simulink model "Wind_Turbine_Modelling"  (R2025a)
settings: Solver=ode23tb  StartTime=0.0  StopTime=1  MaxStep=1e-4  RelTol=1e-3
libraries: simulink x1
settings Model: Creator=Jawad  LastModifiedBy=Jawad

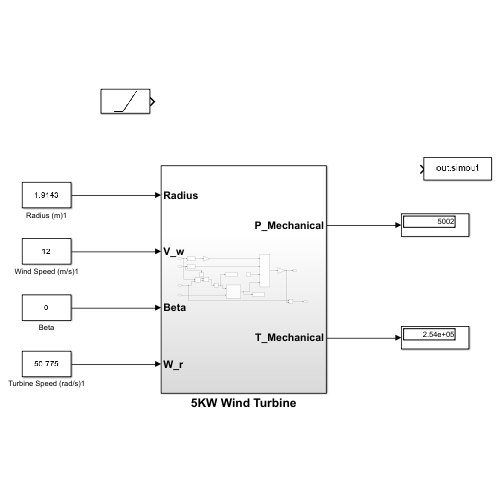
[thumbnail: Simulink's stored preview of the top-level diagram]
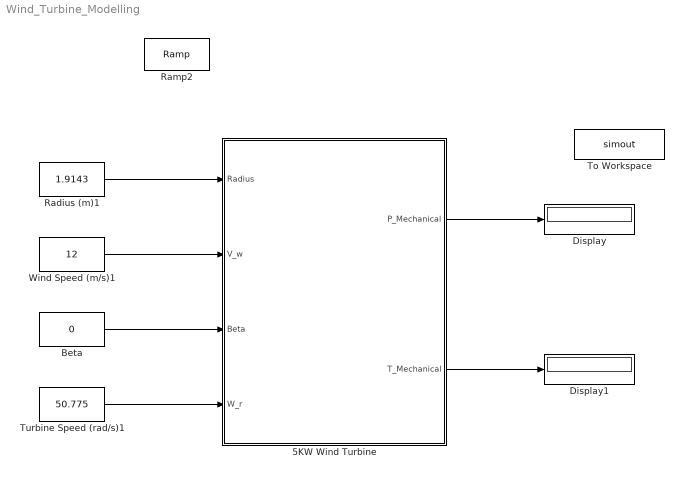
== system Wind_Turbine_Modelling ==
  5KW Wind Turbine : Subsystem
  Beta : Constant  Value=0
  Display : Display
  Display1 : Display
  Radius (m)1 : Constant  Value=1.9143
  Ramp2 : simulink/Sources/Ramp  slope=50  start=0  InitialOutput=0
  To Workspace : ToWorkspace  VariableName=simout  SaveFormat=Timeseries  SampleTime=-1
  Turbine Speed (rad/s)1 : Constant  Value=50.775
  Wind Speed (m/s)1 : Constant  Value=12
  wires:
  Radius (m)1/1 -> 5KW Wind Turbine/1(Radius)
  Wind Speed (m/s)1/1 -> 5KW Wind Turbine/2(V_w)
  Beta/1 -> 5KW Wind Turbine/3(Beta)
  Turbine Speed (rad/s)1/1 -> 5KW Wind Turbine/4(W_r)
  5KW Wind Turbine/1(P_Mechanical) -> Display/1
  5KW Wind Turbine/2(T_Mechanical) -> Display1/1

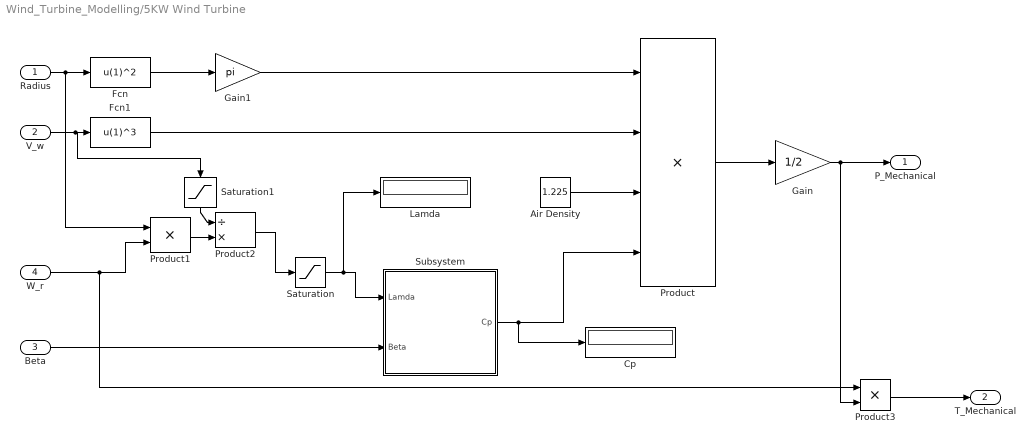
== system Wind_Turbine_Modelling/5KW Wind Turbine ==
  Radius : Inport
  V_w : Inport  Port=2
  Beta : Inport  Port=3
  W_r : Inport  Port=4
  Air Density : Constant  Value=1.225
  Cp : Display
  Fcn : Fcn  Expr=u(1)^2
  Fcn1 : Fcn  Expr=u(1)^3
  Gain : Gain  Gain=1/2
  Gain1 : Gain  Gain=pi
  Lamda : Display
  Product : Product  Inputs=4
  Product1 : Product  Inputs=**
  Product2 : Product  Inputs=/*
  Product3 : Product
  Saturation : Saturate  UpperLimit=inf  LowerLimit=1e-6
  Saturation1 : Saturate  UpperLimit=inf  LowerLimit=1e-6
  Subsystem : Subsystem
  P_Mechanical : Outport
  T_Mechanical : Outport  Port=2
  wires:
  Gain/1 -> Product3/2, P_Mechanical/1
  Product/1 -> Gain/1
  Gain1/1 -> Product/1
  Fcn/1 -> Gain1/1
  Radius/1 -> Product1/1, Fcn/1
  V_w/1 -> Saturation1/1, Fcn1/1
  Fcn1/1 -> Product/2
  Air Density/1 -> Product/3
  Subsystem/1(Cp) -> Cp/1, Product/4
  Beta/1 -> Subsystem/2(Beta)
  W_r/1 -> Product3/1, Product1/2
  Product1/1 -> Product2/2
  Product2/1 -> Saturation/1
  Saturation/1 -> Lamda/1, Subsystem/1(Lamda)
  Saturation1/1 -> Product2/1
  Product3/1 -> T_Mechanical/1

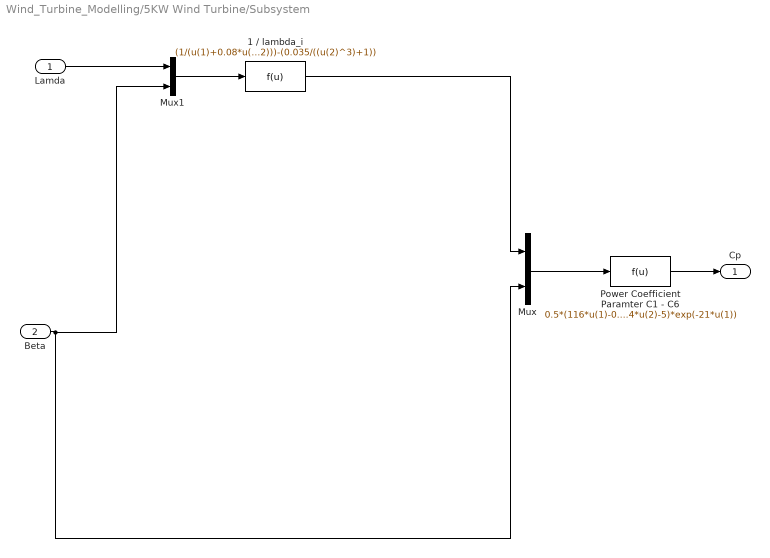
== system Wind_Turbine_Modelling/5KW Wind Turbine/Subsystem ==
  Lamda : Inport
  Beta : Inport  Port=2
  1 / lambda_i : Fcn  Expr=(1/(u(1)+0.08*u(2)))-(0.035/((u(2)^3)+1))
  Mux : Mux  Inputs=2
  Mux1 : Mux  Inputs=2
  Power Coefficient Paramter C1 - C6 : Fcn  Expr=0.5*(116*u(1)-0.4*u(2)-5)*exp(-21*u(1))
  Cp : Outport
  wires:
  Power Coefficient Paramter C1 - C6/1 -> Cp/1
  Mux/1 -> Power Coefficient Paramter C1 - C6/1
  Beta/1 -> Mux1/2, Mux/2
  1 / lambda_i/1 -> Mux/1
  Mux1/1 -> 1 / lambda_i/1
  Lamda/1 -> Mux1/1
